simulink model "Problem3_CruiseControl"  (R2020b)
settings: Solver=VariableStepAuto  StartTime=0.0  StopTime=120  RelTol=1e-3
values from neighbouring files (symbols this model uses):
  b = 50.0    [Data.sldd]
  m = 1000.0    [Data.sldd]
settings Model: DataDictionary=Data.sldd  Creator=vigne  LastModifiedBy=vigne

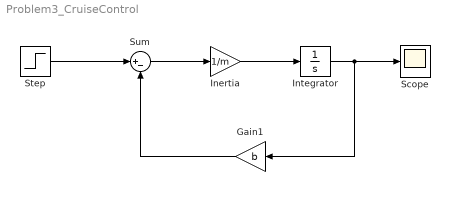
== system Problem3_CruiseControl ==
  Gain1 : Gain  Gain=b
  Inertia : Gain  Gain=1/m
  Integrator : Integrator
  Scope : Scope
  Step : Step  After=u  SampleTime=0
  Sum : Sum  Inputs=|+-
  wires:
  Step/1 -> Sum/1
  Sum/1 -> Inertia/1
  Inertia/1 -> Integrator/1
  Integrator/1 -> Scope/1, Gain1/1
  Gain1/1 -> Sum/2
